simulink model "sm_pto_shaft"  (R2021b)
settings: Solver=ode15s  StartTime=0.0  StopTime=20  MaxStep=0.01  RelTol=1e-6  EnableMultiTasking=on
model workspace: external: MATLAB File sm_pto_shaft_params.m (data not in the file)
undefined symbols (not defined in the file or in its folder): actuator, clamp, linkage, plate, sigbuilder_block, sleeve, X, Y, Z
libraries: sm_lib x147, nesl_utility x8, simulink x1
(part 1 of 4)
Description:
  | Modeling Constant Velocity Joints - PTO Shaft
  | 
  | This example shows a Power Take-Off (PTO) shaft, a device for transferring
  | power from tractor engines to auxiliary equipment such as soil tillers
  | and wood chippers. The model includes two PTO subsystems identical in
  | every sense but their joints. One contains universal (U) joints, the
  | other constant-velocity (CV) joints.
  | 
  | At large bend angles, U joints lead to uneven rotations, subjecting the
  | adjoining shafts to relatively large vibrations and elevated internal
  | stresses. CV joints eliminate these by allowing the shafts to spin at
  | constant velocity, resulting in a smooth motion profile no matter the
  | bend angle.
  | 
  | A single set of motion inputs governs the behavior of the PTO subsystems.
  | The Scope block plots the resulting angular velocities and bend angles of
  | the shafts, enabling you to compare the kinematics of the two joint
  | types.
settings Model: Creator=The MathWorks, Inc.  LastModifiedBy=The MathWorks, Inc.
settings SolverCC: AlgebraicLoopSolver=TrustRegion
settings DataIOCC: LimitDataPoints=on  SaveFormat=Array  ReturnWorkspaceOutputs=off
settings OptimizationCC: LifeSpan=inf
settings DebuggingCC: SolverPrmCheckMsg=warning  SFUnexpectedBacktrackingDiag=warning  SFNoUnconditionalDefaultTransitionDiag=warning  SFExecutionAtInitializationDiag=none  SFMachineParentedDataDiag=warning  ArithmeticOperatorsInVariantConditions=warning
settings HardwareCC: ProdBitPerPointer=32  ProdBitPerSizeT=32  ProdBitPerPtrDiffT=32  ProdLargestAtomicFloat=None  ProdIntDivRoundTo=Undefined  ProdEndianess=Unspecified  ProdWordSize=32  ProdHWDeviceType=32-bit Generic
settings ModelReferenceCC: PropagateSignalLabelsOutOfModel=off
settings SFSimCC: SimUseLocalCustomCode=off  CustomCodeUndefinedFunction=UseInterfaceOnly
settings RTWCC: RTWUseLocalCustomCode=off
settings CodeAppCC: StateflowObjectComments=on
settings GRTTargetCC: TargetLangStandard=C89/C90 (ANSI)
settings ConfigComp: CovMetricSettings=dw  CovSaveCumulativeToWorkspaceVar=on  CovSaveSingleToWorkspaceVar=on  CovExternalEMLEnable=off  CovSFcnEnable=off
settings SimscapeCC: SimscapeNormalizeSystem=off
settings ConfigurationSet: Description=SimMechanics 2G
settings ExplorerConfigSet: InternalSimMechanicsExplorerSettings="<ExplorerConfiguration><canonicalview>default</canonicalview><AnimationSetting><BasePlaybackSpeed>1.0</BasePlaybackSpeed><PlaybackSpeedFactor>1.0</PlaybackSpeedFactor></AnimationSetting><TilePanel><TileInfo><Tiles Columns=\"1\" Count=\"1\" Rows=\"1\"><Column Left=\"2\" Weight=\"1\"/><Column Left=\"821\"/><Row Top=\"2\" Weight=\"1\"/><Row Top=\"584\"/><Tile Height=\"1\" Width=\"1\" X=\"0\" Y=\"0\"/></Tiles></TileInfo><SceneInfo><SceneViewer><BGColor><R>0.60000002384185791</R><G>0.60000002384185791</G><B>0.60000002384185791</B></BGColor><Camera><Position><X>2.5733745767261142</X><Y>-4.7840428425456913</Y><Z>3.9735506250049228</Z></Position><Center><X>-1.2699999809265137</X><Y>-0.94066828489303589</Y><Z>0.13017606735229492</Z></Center><Up><X>-0.40824829046386307</X><Y>0.40824829046386307</Y><Z>0.81649658092772615</Z></Up><Left>-2.0279375195503238</Left><Right>2.0279375195503238</Right><Bottom>-1.7125064849853517</Bottom><Top>1.7125064849853517</Top></Camera></SceneViewer></SceneInfo></TilePanel></ExplorerConfiguration>"

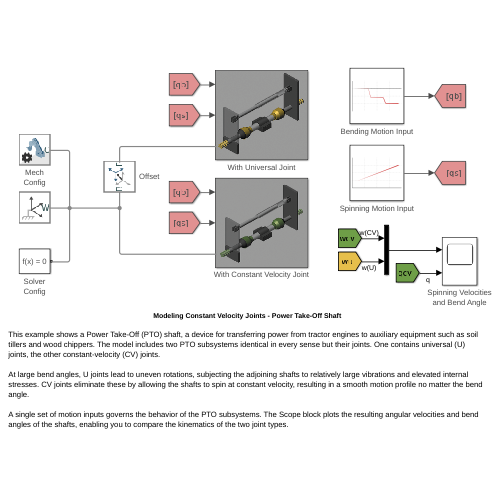
[thumbnail: Simulink's stored preview of the top-level diagram]
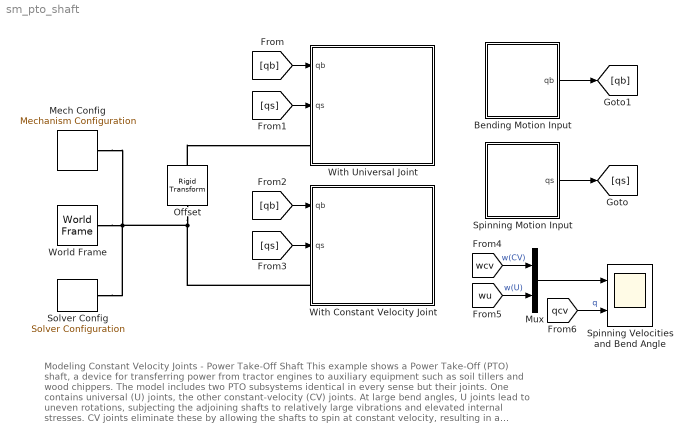
== system sm_pto_shaft ==
  note: Modeling Constant Velocity Joints - Power Take-Off Shaft
      |
      | This example shows a Power Take-Off (PTO) shaft, a device for transferring power from tractor engines to auxiliary equipment such as soil tillers and wood chippers. The model includes two PTO subsystems identical in every sense but their joints. One contains universal (U) joints, the other constant-velocity (CV) joints.
      |
      | At large bend angles, U joints lead to uneven rotations, subjecting the adjoining shafts to relatively large vibrations and elevated internal stresses. CV joints eliminate these by allowing the shafts to spin at constant velocity, resulting in a smooth motion profile no matter the bend angle.
      |
      | A single set of motion inputs governs the behavior of the PTO subsystems. The Scope block plots the resulting angular velocities and bend angles of the shafts, enabling you to compare the kinematics of the two joint types.
  Bending Motion Input : Subsystem
      mask Display: image(fullfile(matlabroot, 'toolbox', 'physmod', 'sm', 'smdemos', 'pto_shaft', 'images', 'bending_signal.svg'));
  Mech Config : sm_lib/Utilities/Mechanism Configuration  UniformGravity=None  GravityVector=[0 0 -9.80665]  GravityUnits=m/s^2  LinearizationDelta=0.001  JointModeTransitionNonlinearIterations=2
  Mux : Mux  Inputs=2
  Offset : sm_lib/Frames and Transforms/Rigid Transform  TranslationMethod=StandardAxis  TranslationStandardOffset=100  TranslationLengthUnit=in  TranslationStandardAxis=-X  TranslationCartesianOffset=[0 0 0]  TranslationROffset=0  TranslationROffsetUnits=m  TranslationZOffset=0  TranslationZOffsetUnits=m  TranslationThetaOffset=0  TranslationThetaOffsetUnits=deg  RotationMethod=None  RotationAngleUnits=deg  RotationStandardAxis=+X  RotationAngle=90  RotationArbitraryAxis=[0 0 1]  FollAlignAxisA=+X  BaseAlignAxisA=+Y  FollAlignAxisB=+Y  BaseAlignAxisB=+Z  RotationSequenceAxes=FollowerAxes  RotationSequence=XYX  RotationSequenceAngles=[0 0 0]  RotationSequenceAnglesUnits=deg  RotationMatrix=[1 0 0; 0 1 0; 0 0 1]
  Solver Config : nesl_utility/Solver Configuration  PhysicalDomain=network_engine_domain  SubClassName=solver  LeftPortType=input  RightPortType=generic  Tones=[]  Harmonics=[]  SimulateNoise=off  Profile=off  UseLocalSampling=off  EnableSwitchedLinearOptims=on  FrequencyDomain=off  UseCCode=off  RelTol=0.001  AbsTol=1e-06  MinStep=1e-09  ToWorkspace=off  RevertToSquareIcSolve=off  NumHomotopyIterations=100  PhasorMode=off  PhasorModeNumHarmonics=1  DoDC=off  ResidualTolerance=1e-09  UseLocalSolver=off  LocalSolverChoice=NE_BACKWARD_EULER_ADVANCER  LocalSolverSampleTime=0.001  DoFixedCost=off  MaxNonlinIter=3  MaxModeIter=2  ComputeImpulses=off  ImpulseIterations=2  LinearAlgebra=Sparse  EquationFormulation=NE_TIME_EF  DelaysMemoryBudget=1024  AutomaticFiltering=on  FilteringTimeConstant=0.001  PartitionStorageMethod=AS_NEEDED  PartitionMemoryBudget=1024  PartitionMethod=FAST
      settings: SourceProductBaseCode=PW,SS
  Spinning Motion Input : Subsystem
      mask Display: image(fullfile(matlabroot, 'toolbox', 'physmod', 'sm', 'smdemos', 'pto_shaft', 'images', 'spinning_ramp.svg'))
  Spinning Velocities and Bend Angle : Scope  NumInputPorts=2
  With Constant Velocity Joint : Subsystem
      mask Display: image(fullfile(matlabroot, 'toolbox', 'physmod', 'sm', 'smdemos', 'pto_shaft', 'images', 'cvj_pto.svg'));
  With Universal Joint : Subsystem
      mask Display: image(fullfile(matlabroot, 'toolbox', 'physmod', 'sm', 'smdemos', 'pto_shaft', 'images', 'uj_pto.svg'));
  World Frame : sm_lib/Frames and Transforms/World Frame
  wires:
  Bending Motion Input/1(qb) -> [qb]
  Spinning Motion Input/1(qs) -> [qs]
  [qb] -> With Constant Velocity Joint/1(qb)
  [qs] -> With Constant Velocity Joint/2(qs)
  [wcv] -> Mux/1  "w(CV)"
  [wu] -> Mux/2  "w(U)"
  Mux/1 -> Spinning Velocities and Bend Angle/1
  [qcv] -> Spinning Velocities and Bend Angle/2  "q"
  [qb] -> With Universal Joint/1(qb)
  [qs] -> With Universal Joint/2(qs)
  connections:
  Offset/RConn1 -- With Universal Joint/LConn1
  Offset/LConn1 -- With Constant Velocity Joint/LConn1 -- Mech Config/RConn1 -- Solver Config/RConn1 -- World Frame/RConn1

== system sm_pto_shaft/Bending Motion Input ==
  Gain : Gain  Gain=14.25
  Nondimensional Actuator Stroke : Subsystem  Tag=STV Subsys  LoadFcn=sigbuilder_block('load');  StartFcn=sigbuilder_block('start');  StopFcn=sigbuilder_block('stop');  ClipboardFcn=sigbuilder_block('clipboard');  mask(Sigbuilder block){tuvar=[0:10]}
      mask help: Simulink:masks:SigbuilderBlock_MD
      mask init:
      | if ~strcmp(get_param(bdroot(gcbh),'SimulationStatus'),'stopped') tuvar = sigbuilder_block('maskInit'); end
      settings: CopyFcn=sigbuilder_block('copy');  DeleteFcn=sigbuilder_block('delete');  ModelCloseFcn=sigbuilder_block('modelClose');  PreSaveFcn=sigbuilder_block('preSave');  PauseFcn=sigbuilder_block('pause');  ContinueFcn=sigbuilder_block('continue');  NameChangeFcn=sigbuilder_block('namechange');  OpenFcn=sigbuilder_block('open',[437.6 199.2 550.4 400 ]);  CloseFcn=sigbuilder_block('close');
      mask Display: plot(0, 0, 100, 100,[2, 2, 32, 32, 2], [68, 8, 8, 68, 68],[32, 2], [38, 38], [32, 19, 2],[53, 60, 44], [32, 17, 17, 2],[16, 16, 31, 31]);txt = getActiveGroup(gcbh);text(2, 100, txt,'verticalAlignment', 'top');
  qb : Outport  VectorParamsAs1DForOutWhenUnconnected=off
  wires:
  Gain/1 -> qb/1
  Nondimensional Actuator Stroke/1(Signal 1) -> Gain/1

== system sm_pto_shaft/Spinning Motion Input ==
  Gain : Gain  Gain=180
  Shaft Rotation : simulink/Sources/Ramp  slope=1  start=1  InitialOutput=0
  qs : Outport  VectorParamsAs1DForOutWhenUnconnected=off
  wires:
  Gain/1 -> qs/1
  Shaft Rotation/1 -> Gain/1

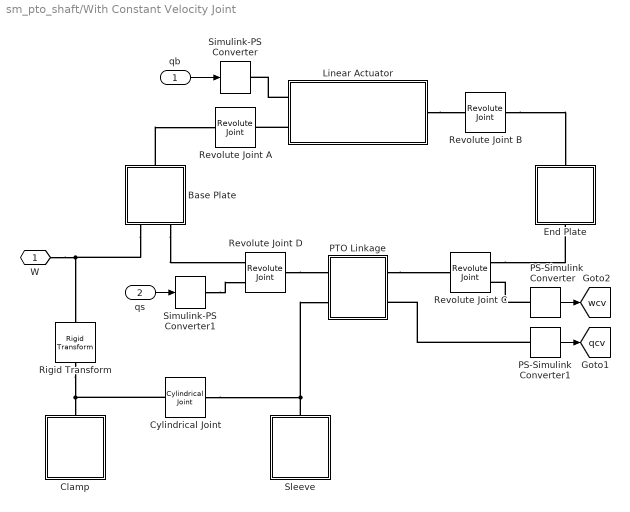
== system sm_pto_shaft/With Constant Velocity Joint ==
  qb : Inport
  qs : Inport  Port=2
  Base Plate : Subsystem  mask(Base Plate){hp=plate.height, wp=plate.width, tp=plate.thickness, R=plate.hole.radius, Lb=plate.bracket.length, wb=plate.bracket.width, tb=plate.bracket.thickness, Ri=plate.bracket.hole.radius, rgb=plate.color, alpha=plate.opacity, rho=plate.density}
      mask prompts: hp "Height (in)"; wp "Width (in)"; tp "Thickness (in)"; R "Hole Radius (in)"; Lb "Length (in)"; wb "Width (in)"; tb "Thickness (in)"; Ri "Inner Radius (in)"; rgb "Color (RGB)"; alpha "Opacity (unitless)"; rho "Density (kg/m^3)"
      mask help: This block models the fixed base plate supporting the PTO linkage.
      mask init:
      | % Plate cross-section coordinates:
      | theta = linspace(0, -pi)';
      | plateBottomCS = [-wp/2 -hp/4; wp/2 -hp/4; wp/2 0; R*cos(theta) R*sin(theta); -wp/2 0];
      | theta = linspace(pi, 0)';
      | plateTopCS = [-wp/2 0; R*cos(theta) R*sin(theta); wp/2 0; wp/2 3*hp/4; -wp/2 3*hp/4];
      | 
      | % Bracket cross-section coordinates:
      | Ro = wb/2;
      | theta = linspace(3*pi/2, pi/2)';
      | bracketBottomCS = [0 wb/2; -Lb wb/2; -Lb -wb/2; 0 -wb/2; Ri*cos(theta) Ri*sin(theta)];
      | thetaA = linspace(-pi/2, pi/2)';
      | betaB = linspace(pi/2, -pi/2)';
      | bracketTopCS = [Ro*cos(thetaA) Ro*sin(thetaA); Ri*cos(betaB) Ri*sin(betaB)];
      mask DialogControl Container19 Prompt: Plate
      mask DialogControl Container15 Prompt: Bracket
      mask DialogControl Container16 Prompt: Material Properties
      mask Display: image(fullfile(matlabroot, 'toolbox', 'physmod', 'sm', 'smdemos', 'pto_shaft', 'images', 'base.png'));
  Clamp : Subsystem  mask(Clamp){L=clamp.length, T=clamp.thickness, R=clamp.radius, D=clamp.wing.width, rgbClamp=clamp.color, rho=clamp.density}
      mask prompts: L "Length (in)"; T "Wall Thickness (in)"; R "Hole Radius (in)"; D "Wing Width (in)"; rgbClamp "Color (RGB)"; rho "Density (kg/m^3)"
      mask help: This block models a clamp used to hold the central shaft of the PTO linkage fixed.
      mask init:
      | % Common Parameters
      | HW = R+T+D; % Clamp Half Width
      | Ro = R + T; % Outer Clamp Radius
      | 
      | % Bottom Half CS
      | theta = linspace(0, -pi)';
      | bottomCS = [-HW -Ro; HW -Ro; HW 0; ...
      |     R*cos(theta) R*sin(theta); -HW 0];
      | 
      | % Top Half CS
      | theta = linspace(pi, 0)';
      | alpha = linspace(asin(T/Ro), pi-asin(T/Ro))';
      | topCS = [-HW 0; R*cos(theta) R*sin(theta); HW 0; HW T; ...
      |     Ro*cos(alpha) Ro*sin(alpha); -HW T];
      mask Display: image(fullfile(matlabroot, 'toolbox', 'physmod', 'sm', 'smdemos', 'pto_shaft', 'images', 'clamp.png'));
  Cylindrical Joint : sm_lib/Joints/Cylindrical Joint  JointMode=Normal  SenseConstraintForce=off  SenseConstraintForceX=off  SenseConstraintForceY=off  SenseConstraintForceZ=off  SenseConstraintTorque=off  SenseConstraintTorqueX=off  SenseConstraintTorqueY=off  SenseConstraintTorqueZ=off  SenseTotalForce=off  SenseTotalForceX=off  SenseTotalForceY=off  SenseTotalForceZ=off  SenseTotalTorque=off  SenseTotalTorqueX=off  SenseTotalTorqueY=off  SenseTotalTorqueZ=off  CompositeWrenchDir=FollowerOnBase  CompositeWrenchFrame=BaseFrame  PzEquilibriumPosition=0  PzEquilibriumPositionUnits=m  PzSpringStiffness=0  PzSpringStiffnessUnits=N/m  PzDampingCoefficient=0  PzDampingCoefficientUnits=N/(m/s)  PzTorqueActuationMode=NoTorque  PzMotionActuationMode=ComputedMotion  PzSensePosition=off  PzSenseVelocity=off  PzSenseAcceleration=off  PzSenseTorqueForce=off  PzSenseLowerLimitTorqueForce=off  PzSenseUpperLimitTorqueForce=off  PzLowerLimitSpecify=off  PzLowerLimitBound=-1  PzLowerLimitBoundUnits=m  PzLowerLimitStiffness=1e6  PzLowerLimitStiffnessUnits=N/m  PzLowerLimitDamping=1e3  PzLowerLimitDampingUnits=N/(m/s)  PzLowerLimitTransitionRegionWidth=1e-4  PzLowerLimitTransitionRegionWidthUnits=m  PzUpperLimitSpecify=off  PzUpperLimitBound=1  PzUpperLimitBoundUnits=m  PzUpperLimitStiffness=1e6  PzUpperLimitStiffnessUnits=N/m  PzUpperLimitDamping=1e3  PzUpperLimitDampingUnits=N/(m/s)  PzUpperLimitTransitionRegionWidth=1e-4  PzUpperLimitTransitionRegionWidthUnits=m  PzPositionTargetSpecify=off  PzPositionTargetPriority=High  PzPositionTargetValue=0  PzPositionTargetValueUnits=m  PzVelocityTargetSpecify=off  PzVelocityTargetPriority=High  PzVelocityTargetValue=0  PzVelocityTargetValueUnits=m/s  RzEquilibriumPosition=0  RzEquilibriumPositionUnits=deg  RzSpringStiffness=0  RzSpringStiffnessUnits=N*m/deg  RzDampingCoefficient=0  RzDampingCoefficientUnits=N*m/(deg/s)  RzTorqueActuationMode=NoTorque  RzMotionActuationMode=ComputedMotion  RzSensePosition=off  RzSenseVelocity=off  RzSenseAcceleration=off  RzSenseTorqueForce=off  RzSenseLowerLimitTorqueForce=off  RzSenseUpperLimitTorqueForce=off  RzLowerLimitSpecify=off  RzLowerLimitBound=-90  RzLowerLimitBoundUnits=deg  RzLowerLimitStiffness=1e4  RzLowerLimitStiffnessUnits=N*m/deg  RzLowerLimitDamping=10  RzLowerLimitDampingUnits=N*m/(deg/s)  RzLowerLimitTransitionRegionWidth=0.1  RzLowerLimitTransitionRegionWidthUnits=deg  RzUpperLimitSpecify=off  RzUpperLimitBound=90  RzUpperLimitBoundUnits=deg  RzUpperLimitStiffness=1e4  RzUpperLimitStiffnessUnits=N*m/deg  RzUpperLimitDamping=10  RzUpperLimitDampingUnits=N*m/(deg/s)  RzUpperLimitTransitionRegionWidth=0.1  RzUpperLimitTransitionRegionWidthUnits=deg  RzPositionTargetSpecify=off  RzPositionTargetPriority=High  RzPositionTargetValue=0  RzPositionTargetValueUnits=deg  RzVelocityTargetSpecify=off  RzVelocityTargetPriority=High  RzVelocityTargetValue=0  RzVelocityTargetValueUnits=deg/s
  End Plate : Subsystem  mask(End Plate){hp=plate.height, wp=plate.width, tp=plate.thickness, R=plate.hole.radius, Lb=plate.bracket.length, wb=plate.bracket.width, tb=plate.bracket.thickness, Ri=plate.bracket.hole.radius, rgb=plate.color, alpha=plate.opacity, rho=plate.density}
      mask prompts: hp "Height (in)"; wp "Width (in)"; tp "Thickness (in)"; R "Hole Radius (in)"; Lb "Length (in)"; wb "Width (in)"; tb "Thickness (in)"; Ri "Inner Radius (in)"; rgb "Color (RGB)"; alpha "Opacity (unitless)"; rho "Density (kg/m^3)"
      mask help: This block models the tilting end plate supporting the PTO linkage.
      mask init: same as sm_pto_shaft/With Constant Velocity Joint/Base Plate
      mask DialogControl Container19 Prompt: Plate
      mask DialogControl Container15 Prompt: Bracket
      mask DialogControl Container16 Prompt: Material Properties
      mask Display: image(fullfile(matlabroot, 'toolbox', 'physmod', 'sm', 'smdemos', 'pto_shaft', 'images', 'base.png'));
  Linear Actuator : Subsystem
      mask Display: image(fullfile(matlabroot, 'toolbox', 'physmod', 'sm', 'smdemos', 'pto_shaft', 'images', 'linear_actuator.png'));
  PS-Simulink Converter : nesl_utility/PS-Simulink Converter  PhysicalDomain=network_engine_domain  SubClassName=ps_output  LeftPortType=input  RightPortType=output  PseudoPeriodic=off  Frequencies=[]  Unit=deg/s  AffineConversion=off
      settings: SourceProductBaseCode=PW,SS
  PS-Simulink Converter1 : nesl_utility/PS-Simulink Converter  PhysicalDomain=network_engine_domain  SubClassName=ps_output  LeftPortType=input  RightPortType=output  PseudoPeriodic=off  Frequencies=[]  Unit=deg  AffineConversion=off
      settings: SourceProductBaseCode=PW,SS
  PTO Linkage : Subsystem
      mask Display: image(fullfile(matlabroot, 'toolbox', 'physmod', 'sm', 'smdemos', 'pto_shaft', 'images', 'pto_linkage.png'));
  Revolute Joint A : sm_lib/Joints/Revolute Joint  JointMode=Normal  SenseConstraintForce=off  SenseConstraintForceX=off  SenseConstraintForceY=off  SenseConstraintForceZ=off  SenseConstraintTorque=off  SenseConstraintTorqueX=off  SenseConstraintTorqueY=off  SenseConstraintTorqueZ=off  SenseTotalForce=off  SenseTotalForceX=off  SenseTotalForceY=off  SenseTotalForceZ=off  SenseTotalTorque=off  SenseTotalTorqueX=off  SenseTotalTorqueY=off  SenseTotalTorqueZ=off  CompositeWrenchDir=FollowerOnBase  CompositeWrenchFrame=BaseFrame  EquilibriumPosition=0  EquilibriumPositionUnits=deg  SpringStiffness=0  SpringStiffnessUnits=N*m/deg  DampingCoefficient=0  DampingCoefficientUnits=N*m/(deg/s)  TorqueActuationMode=NoTorque  MotionActuationMode=ComputedMotion  SensePosition=off  SenseVelocity=off  SenseAcceleration=off  SenseTorqueForce=off  SenseLowerLimitTorqueForce=off  SenseUpperLimitTorqueForce=off  LowerLimitSpecify=off  LowerLimitBound=-90  LowerLimitBoundUnits=deg  LowerLimitStiffness=1e4  LowerLimitStiffnessUnits=N*m/deg  LowerLimitDamping=10  LowerLimitDampingUnits=N*m/(deg/s)  LowerLimitTransitionRegionWidth=0.1  LowerLimitTransitionRegionWidthUnits=deg  UpperLimitSpecify=off  UpperLimitBound=90  UpperLimitBoundUnits=deg  UpperLimitStiffness=1e4  UpperLimitStiffnessUnits=N*m/deg  UpperLimitDamping=10  UpperLimitDampingUnits=N*m/(deg/s)  UpperLimitTransitionRegionWidth=0.1  UpperLimitTransitionRegionWidthUnits=deg  PositionTargetSpecify=off  PositionTargetPriority=High  PositionTargetValue=0  PositionTargetValueUnits=deg  VelocityTargetSpecify=off  VelocityTargetPriority=High  VelocityTargetValue=0  VelocityTargetValueUnits=deg/s
  Revolute Joint B : sm_lib/Joints/Revolute Joint  JointMode=Normal  SenseConstraintForce=off  SenseConstraintForceX=off  SenseConstraintForceY=off  SenseConstraintForceZ=off  SenseConstraintTorque=off  SenseConstraintTorqueX=off  SenseConstraintTorqueY=off  SenseConstraintTorqueZ=off  SenseTotalForce=off  SenseTotalForceX=off  SenseTotalForceY=off  SenseTotalForceZ=off  SenseTotalTorque=off  SenseTotalTorqueX=off  SenseTotalTorqueY=off  SenseTotalTorqueZ=off  CompositeWrenchDir=FollowerOnBase  CompositeWrenchFrame=BaseFrame  EquilibriumPosition=0  EquilibriumPositionUnits=deg  SpringStiffness=0  SpringStiffnessUnits=N*m/deg  DampingCoefficient=0  DampingCoefficientUnits=N*m/(deg/s)  TorqueActuationMode=NoTorque  MotionActuationMode=ComputedMotion  SensePosition=off  SenseVelocity=off  SenseAcceleration=off  SenseTorqueForce=off  SenseLowerLimitTorqueForce=off  SenseUpperLimitTorqueForce=off  LowerLimitSpecify=off  LowerLimitBound=-90  LowerLimitBoundUnits=deg  LowerLimitStiffness=1e4  LowerLimitStiffnessUnits=N*m/deg  LowerLimitDamping=10  LowerLimitDampingUnits=N*m/(deg/s)  LowerLimitTransitionRegionWidth=0.1  LowerLimitTransitionRegionWidthUnits=deg  UpperLimitSpecify=off  UpperLimitBound=90  UpperLimitBoundUnits=deg  UpperLimitStiffness=1e4  UpperLimitStiffnessUnits=N*m/deg  UpperLimitDamping=10  UpperLimitDampingUnits=N*m/(deg/s)  UpperLimitTransitionRegionWidth=0.1  UpperLimitTransitionRegionWidthUnits=deg  PositionTargetSpecify=off  PositionTargetPriority=High  PositionTargetValue=0  PositionTargetValueUnits=deg  VelocityTargetSpecify=off  VelocityTargetPriority=High  VelocityTargetValue=0  VelocityTargetValueUnits=deg/s
  Revolute Joint C : sm_lib/Joints/Revolute Joint  JointMode=Normal  SenseConstraintForce=off  SenseConstraintForceX=off  SenseConstraintForceY=off  SenseConstraintForceZ=off  SenseConstraintTorque=off  SenseConstraintTorqueX=off  SenseConstraintTorqueY=off  SenseConstraintTorqueZ=off  SenseTotalForce=off  SenseTotalForceX=off  SenseTotalForceY=off  SenseTotalForceZ=off  SenseTotalTorque=off  SenseTotalTorqueX=off  SenseTotalTorqueY=off  SenseTotalTorqueZ=off  CompositeWrenchDir=FollowerOnBase  CompositeWrenchFrame=BaseFrame  EquilibriumPosition=0  EquilibriumPositionUnits=deg  SpringStiffness=0  SpringStiffnessUnits=N*m/deg  DampingCoefficient=0  DampingCoefficientUnits=N*m/(deg/s)  TorqueActuationMode=NoTorque  MotionActuationMode=ComputedMotion  SensePosition=off  SenseVelocity=on  SenseAcceleration=off  SenseTorqueForce=off  SenseLowerLimitTorqueForce=off  SenseUpperLimitTorqueForce=off  LowerLimitSpecify=off  LowerLimitBound=-90  LowerLimitBoundUnits=deg  LowerLimitStiffness=1e4  LowerLimitStiffnessUnits=N*m/deg  LowerLimitDamping=10  LowerLimitDampingUnits=N*m/(deg/s)  LowerLimitTransitionRegionWidth=0.1  LowerLimitTransitionRegionWidthUnits=deg  UpperLimitSpecify=off  UpperLimitBound=90  UpperLimitBoundUnits=deg  UpperLimitStiffness=1e4  UpperLimitStiffnessUnits=N*m/deg  UpperLimitDamping=10  UpperLimitDampingUnits=N*m/(deg/s)  UpperLimitTransitionRegionWidth=0.1  UpperLimitTransitionRegionWidthUnits=deg  PositionTargetSpecify=off  PositionTargetPriority=High  PositionTargetValue=0  PositionTargetValueUnits=deg  VelocityTargetSpecify=off  VelocityTargetPriority=High  VelocityTargetValue=0  VelocityTargetValueUnits=deg/s
  Revolute Joint D : sm_lib/Joints/Revolute Joint  JointMode=Normal  SenseConstraintForce=off  SenseConstraintForceX=off  SenseConstraintForceY=off  SenseConstraintForceZ=off  SenseConstraintTorque=off  SenseConstraintTorqueX=off  SenseConstraintTorqueY=off  SenseConstraintTorqueZ=off  SenseTotalForce=off  SenseTotalForceX=off  SenseTotalForceY=off  SenseTotalForceZ=off  SenseTotalTorque=off  SenseTotalTorqueX=off  SenseTotalTorqueY=off  SenseTotalTorqueZ=off  CompositeWrenchDir=FollowerOnBase  CompositeWrenchFrame=BaseFrame  EquilibriumPosition=0  EquilibriumPositionUnits=deg  SpringStiffness=0  SpringStiffnessUnits=N*m/deg  DampingCoefficient=0  DampingCoefficientUnits=N*m/(deg/s)  TorqueActuationMode=ComputedTorque  MotionActuationMode=InputMotion  SensePosition=off  SenseVelocity=off  SenseAcceleration=off  SenseTorqueForce=off  SenseLowerLimitTorqueForce=off  SenseUpperLimitTorqueForce=off  LowerLimitSpecify=off  LowerLimitBound=-90  LowerLimitBoundUnits=deg  LowerLimitStiffness=1e4  LowerLimitStiffnessUnits=N*m/deg  LowerLimitDamping=10  LowerLimitDampingUnits=N*m/(deg/s)  LowerLimitTransitionRegionWidth=0.1  LowerLimitTransitionRegionWidthUnits=deg  UpperLimitSpecify=off  UpperLimitBound=90  UpperLimitBoundUnits=deg  UpperLimitStiffness=1e4  UpperLimitStiffnessUnits=N*m/deg  UpperLimitDamping=10  UpperLimitDampingUnits=N*m/(deg/s)  UpperLimitTransitionRegionWidth=0.1  UpperLimitTransitionRegionWidthUnits=deg  PositionTargetSpecify=off  PositionTargetPriority=High  PositionTargetValue=0  PositionTargetValueUnits=deg  VelocityTargetSpecify=off  VelocityTargetPriority=High  VelocityTargetValue=0  VelocityTargetValueUnits=deg/s
  Rigid Transform : sm_lib/Frames and Transforms/Rigid Transform  TranslationMethod=StandardAxis  TranslationStandardOffset=34  TranslationLengthUnit=in  TranslationStandardAxis=-Y  TranslationCartesianOffset=[0 0 0]  TranslationROffset=0  TranslationROffsetUnits=m  TranslationZOffset=0  TranslationZOffsetUnits=m  TranslationThetaOffset=0  TranslationThetaOffsetUnits=deg  RotationMethod=StandardAxis  RotationAngleUnits=deg  RotationStandardAxis=+X  RotationAngle=90  RotationArbitraryAxis=[0 0 1]  FollAlignAxisA=+X  BaseAlignAxisA=+Y  FollAlignAxisB=+Y  BaseAlignAxisB=+Z  RotationSequenceAxes=FollowerAxes  RotationSequence=XYX  RotationSequenceAngles=[0 0 0]  RotationSequenceAnglesUnits=deg  RotationMatrix=[1 0 0; 0 1 0; 0 0 1]
  Simulink-PS Converter : nesl_utility/Simulink-PS Converter  PhysicalDomain=network_engine_domain  SubClassName=ps_input  LeftPortType=input  RightPortType=output  PseudoPeriodic=off  Frequencies=[]  NoiseDistribution=none  NoiseParameters=[]  Unit=in  AffineConversion=off  FilteringAndDerivatives=filter  SimscapeFilterOrder=2  InputFilterTimeConstant=0.1  UdotUserProvided=1
      settings: SourceProductBaseCode=PW,SS
  Simulink-PS Converter1 : nesl_utility/Simulink-PS Converter  PhysicalDomain=network_engine_domain  SubClassName=ps_input  LeftPortType=input  RightPortType=output  PseudoPeriodic=off  Frequencies=[]  NoiseDistribution=none  NoiseParameters=[]  Unit=deg  AffineConversion=off  FilteringAndDerivatives=filter  SimscapeFilterOrder=2  InputFilterTimeConstant=0.01  UdotUserProvided=1
      settings: SourceProductBaseCode=PW,SS
  Sleeve : Subsystem  mask(Sleeve){L=sleeve.length, R=sleeve.radius, t=sleeve.thickness, rgbShaft=sleeve.colorA, rgbBoot=sleeve.colorCVJ, rho=sleeve.density}
      mask prompts: L "Shaft Length (in)"; R "Shaft Radius (in)"; t "Shaft Thickness (in)"; rgbShaft "Shaft Color (RGB)"; rgbBoot "Boot Color (RGB)"; rho "Density (kg/m^3)"
      mask help: This block models a sleeve covering the central shaft of the PTO linkage.
      mask init:
      | bootCS = [2.77 0;2.77 0.22;2.66 0.22;2.66 2.33;3.33 2.33;4.55 4.77;4.77 9.5;4.22 4.77;3.11 2.66;2.44 2.66;2.44 0.33;1.44 0.33;1.44 0];
      | shaftCS = [(R-t) -L/2; R -L/2; R L/2; (R-t) L/2];
      mask Display: image(fullfile(matlabroot, 'toolbox', 'physmod', 'sm', 'smdemos', 'pto_shaft', 'images', 'cvj_sleeve.png'));
  W : PMIOPort  Side=Left
  tag scope: qcv=global, wcv=global
  wires:
  qb/1 -> Simulink-PS Converter/1
  qs/1 -> Simulink-PS Converter1/1
  PS-Simulink Converter/1 -> [wcv]
  PS-Simulink Converter1/1 -> [qcv]
  connections:
  Linear Actuator/LConn1 -- Simulink-PS Converter/RConn1
  Rigid Transform/RConn1 -- Clamp/RConn1 -- Cylindrical Joint/LConn1
  W/RConn1 -- Base Plate/LConn1 -- Rigid Transform/LConn1
  Sleeve/LConn1 -- PTO Linkage/RConn2 -- Cylindrical Joint/RConn1
  Linear Actuator/RConn1 -- Revolute Joint B/LConn1
  Linear Actuator/LConn2 -- Revolute Joint A/RConn1
  Simulink-PS Converter1/RConn1 -- Revolute Joint D/LConn2
  PS-Simulink Converter/LConn1 -- Revolute Joint C/RConn2
  Revolute Joint C/RConn1 -- End Plate/LConn1
  Revolute Joint B/RConn1 -- End Plate/RConn1
  Base Plate/RConn1 -- Revolute Joint A/LConn1
  Base Plate/LConn2 -- Revolute Joint D/LConn1
  Revolute Joint D/RConn1 -- PTO Linkage/RConn1
  PTO Linkage/LConn1 -- Revolute Joint C/LConn1
  PS-Simulink Converter1/LConn1 -- PTO Linkage/LConn2

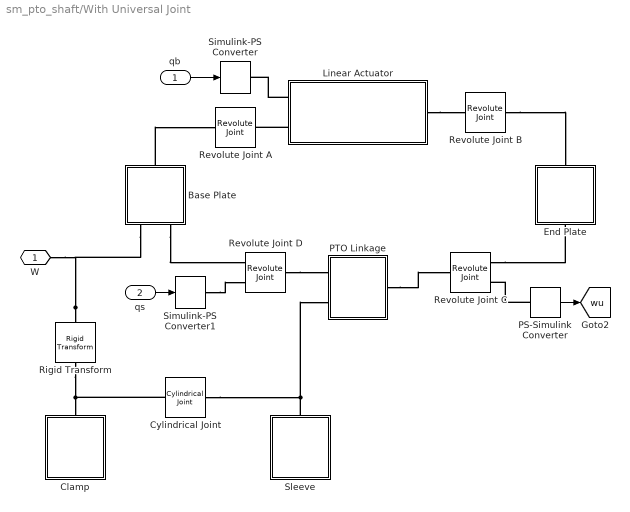
== system sm_pto_shaft/With Universal Joint ==
  qb : Inport
  qs : Inport  Port=2
  Base Plate : Subsystem  mask(Base Plate){hp=plate.height, wp=plate.width, tp=plate.thickness, R=plate.hole.radius, Lb=plate.bracket.length, wb=plate.bracket.width, tb=plate.bracket.thickness, Ri=plate.bracket.hole.radius, rgb=plate.color, alpha=plate.opacity, rho=plate.density}
      mask prompts: hp "Height (in)"; wp "Width (in)"; tp "Thickness (in)"; R "Hole Radius (in)"; Lb "Length (in)"; wb "Width (in)"; tb "Thickness (in)"; Ri "Inner Radius (in)"; rgb "Color (RGB)"; alpha "Opacity (unitless)"; rho "Density (kg/m^3)"
      mask help: This block models the fixed base plate supporting the PTO linkage.
      mask init: same as sm_pto_shaft/With Constant Velocity Joint/Base Plate
      mask DialogControl Container19 Prompt: Plate
      mask DialogControl Container15 Prompt: Bracket
      mask DialogControl Container16 Prompt: Material Properties
      mask Display: image(fullfile(matlabroot, 'toolbox', 'physmod', 'sm', 'smdemos', 'pto_shaft', 'images', 'base.png'));
  Clamp : Subsystem  mask(Clamp){L=clamp.length, T=clamp.thickness, R=clamp.radius, D=clamp.wing.width, rgbClamp=clamp.color, rho=clamp.density}
      mask prompts: L "Length (in)"; T "Wall Thickness (in)"; R "Hole Radius (in)"; D "Wing Width (in)"; rgbClamp "Color (RGB)"; rho "Density (kg/m^3)"
      mask help: This block models a clamp used to hold the central shaft of the PTO linkage fixed.
      mask init: same as sm_pto_shaft/With Constant Velocity Joint/Clamp
      mask Display: image(fullfile(matlabroot, 'toolbox', 'physmod', 'sm', 'smdemos', 'pto_shaft', 'images', 'clamp.png'));
  Cylindrical Joint : sm_lib/Joints/Cylindrical Joint  JointMode=Normal  SenseConstraintForce=off  SenseConstraintForceX=off  SenseConstraintForceY=off  SenseConstraintForceZ=off  SenseConstraintTorque=off  SenseConstraintTorqueX=off  SenseConstraintTorqueY=off  SenseConstraintTorqueZ=off  SenseTotalForce=off  SenseTotalForceX=off  SenseTotalForceY=off  SenseTotalForceZ=off  SenseTotalTorque=off  SenseTotalTorqueX=off  SenseTotalTorqueY=off  SenseTotalTorqueZ=off  CompositeWrenchDir=FollowerOnBase  CompositeWrenchFrame=BaseFrame  PzEquilibriumPosition=0  PzEquilibriumPositionUnits=m  PzSpringStiffness=0  PzSpringStiffnessUnits=N/m  PzDampingCoefficient=0  PzDampingCoefficientUnits=N/(m/s)  PzTorqueActuationMode=NoTorque  PzMotionActuationMode=ComputedMotion  PzSensePosition=off  PzSenseVelocity=off  PzSenseAcceleration=off  PzSenseTorqueForce=off  PzSenseLowerLimitTorqueForce=off  PzSenseUpperLimitTorqueForce=off  PzLowerLimitSpecify=off  PzLowerLimitBound=-1  PzLowerLimitBoundUnits=m  PzLowerLimitStiffness=1e6  PzLowerLimitStiffnessUnits=N/m  PzLowerLimitDamping=1e3  PzLowerLimitDampingUnits=N/(m/s)  PzLowerLimitTransitionRegionWidth=1e-4  PzLowerLimitTransitionRegionWidthUnits=m  PzUpperLimitSpecify=off  PzUpperLimitBound=1  PzUpperLimitBoundUnits=m  PzUpperLimitStiffness=1e6  PzUpperLimitStiffnessUnits=N/m  PzUpperLimitDamping=1e3  PzUpperLimitDampingUnits=N/(m/s)  PzUpperLimitTransitionRegionWidth=1e-4  PzUpperLimitTransitionRegionWidthUnits=m  PzPositionTargetSpecify=off  PzPositionTargetPriority=High  PzPositionTargetValue=0  PzPositionTargetValueUnits=m  PzVelocityTargetSpecify=off  PzVelocityTargetPriority=High  PzVelocityTargetValue=0  PzVelocityTargetValueUnits=m/s  RzEquilibriumPosition=0  RzEquilibriumPositionUnits=deg  RzSpringStiffness=0  RzSpringStiffnessUnits=N*m/deg  RzDampingCoefficient=0  RzDampingCoefficientUnits=N*m/(deg/s)  RzTorqueActuationMode=NoTorque  RzMotionActuationMode=ComputedMotion  RzSensePosition=off  RzSenseVelocity=off  RzSenseAcceleration=off  RzSenseTorqueForce=off  RzSenseLowerLimitTorqueForce=off  RzSenseUpperLimitTorqueForce=off  RzLowerLimitSpecify=off  RzLowerLimitBound=-90  RzLowerLimitBoundUnits=deg  RzLowerLimitStiffness=1e4  RzLowerLimitStiffnessUnits=N*m/deg  RzLowerLimitDamping=10  RzLowerLimitDampingUnits=N*m/(deg/s)  RzLowerLimitTransitionRegionWidth=0.1  RzLowerLimitTransitionRegionWidthUnits=deg  RzUpperLimitSpecify=off  RzUpperLimitBound=90  RzUpperLimitBoundUnits=deg  RzUpperLimitStiffness=1e4  RzUpperLimitStiffnessUnits=N*m/deg  RzUpperLimitDamping=10  RzUpperLimitDampingUnits=N*m/(deg/s)  RzUpperLimitTransitionRegionWidth=0.1  RzUpperLimitTransitionRegionWidthUnits=deg  RzPositionTargetSpecify=off  RzPositionTargetPriority=High  RzPositionTargetValue=0  RzPositionTargetValueUnits=deg  RzVelocityTargetSpecify=off  RzVelocityTargetPriority=High  RzVelocityTargetValue=0  RzVelocityTargetValueUnits=deg/s
  End Plate : Subsystem  mask(End Plate){hp=plate.height, wp=plate.width, tp=plate.thickness, R=plate.hole.radius, Lb=plate.bracket.length, wb=plate.bracket.width, tb=plate.bracket.thickness, Ri=plate.bracket.hole.radius, rgb=plate.color, alpha=plate.opacity, rho=plate.density}
      mask prompts: hp "Height (in)"; wp "Width (in)"; tp "Thickness (in)"; R "Hole Radius (in)"; Lb "Length (in)"; wb "Width (in)"; tb "Thickness (in)"; Ri "Inner Radius (in)"; rgb "Color (RGB)"; alpha "Opacity (unitless)"; rho "Density (kg/m^3)"
      mask help: This block models the tilting end plate supporting the PTO linkage.
      mask init: same as sm_pto_shaft/With Constant Velocity Joint/Base Plate
      mask DialogControl Container19 Prompt: Plate
      mask DialogControl Container15 Prompt: Bracket
      mask DialogControl Container16 Prompt: Material Properties
      mask Display: image(fullfile(matlabroot, 'toolbox', 'physmod', 'sm', 'smdemos', 'pto_shaft', 'images', 'base.png'));
  Linear Actuator : Subsystem
      mask Display: image(fullfile(matlabroot, 'toolbox', 'physmod', 'sm', 'smdemos', 'pto_shaft', 'images', 'linear_actuator.png'));
  PS-Simulink Converter : nesl_utility/PS-Simulink Converter  PhysicalDomain=network_engine_domain  SubClassName=ps_output  LeftPortType=input  RightPortType=output  PseudoPeriodic=off  Frequencies=[]  Unit=deg/s  AffineConversion=off
      settings: SourceProductBaseCode=PW,SS
  PTO Linkage : Subsystem
      mask Display: image(fullfile(matlabroot, 'toolbox', 'physmod', 'sm', 'smdemos', 'pto_shaft', 'images', 'pto_linkage.png'));
  Revolute Joint A : sm_lib/Joints/Revolute Joint  JointMode=Normal  SenseConstraintForce=off  SenseConstraintForceX=off  SenseConstraintForceY=off  SenseConstraintForceZ=off  SenseConstraintTorque=off  SenseConstraintTorqueX=off  SenseConstraintTorqueY=off  SenseConstraintTorqueZ=off  SenseTotalForce=off  SenseTotalForceX=off  SenseTotalForceY=off  SenseTotalForceZ=off  SenseTotalTorque=off  SenseTotalTorqueX=off  SenseTotalTorqueY=off  SenseTotalTorqueZ=off  CompositeWrenchDir=FollowerOnBase  CompositeWrenchFrame=BaseFrame  EquilibriumPosition=0  EquilibriumPositionUnits=deg  SpringStiffness=0  SpringStiffnessUnits=N*m/deg  DampingCoefficient=0  DampingCoefficientUnits=N*m/(deg/s)  TorqueActuationMode=NoTorque  MotionActuationMode=ComputedMotion  SensePosition=off  SenseVelocity=off  SenseAcceleration=off  SenseTorqueForce=off  SenseLowerLimitTorqueForce=off  SenseUpperLimitTorqueForce=off  LowerLimitSpecify=off  LowerLimitBound=-90  LowerLimitBoundUnits=deg  LowerLimitStiffness=1e4  LowerLimitStiffnessUnits=N*m/deg  LowerLimitDamping=10  LowerLimitDampingUnits=N*m/(deg/s)  LowerLimitTransitionRegionWidth=0.1  LowerLimitTransitionRegionWidthUnits=deg  UpperLimitSpecify=off  UpperLimitBound=90  UpperLimitBoundUnits=deg  UpperLimitStiffness=1e4  UpperLimitStiffnessUnits=N*m/deg  UpperLimitDamping=10  UpperLimitDampingUnits=N*m/(deg/s)  UpperLimitTransitionRegionWidth=0.1  UpperLimitTransitionRegionWidthUnits=deg  PositionTargetSpecify=off  PositionTargetPriority=High  PositionTargetValue=0  PositionTargetValueUnits=deg  VelocityTargetSpecify=off  VelocityTargetPriority=High  VelocityTargetValue=0  VelocityTargetValueUnits=deg/s
  Revolute Joint B : sm_lib/Joints/Revolute Joint  JointMode=Normal  SenseConstraintForce=off  SenseConstraintForceX=off  SenseConstraintForceY=off  SenseConstraintForceZ=off  SenseConstraintTorque=off  SenseConstraintTorqueX=off  SenseConstraintTorqueY=off  SenseConstraintTorqueZ=off  SenseTotalForce=off  SenseTotalForceX=off  SenseTotalForceY=off  SenseTotalForceZ=off  SenseTotalTorque=off  SenseTotalTorqueX=off  SenseTotalTorqueY=off  SenseTotalTorqueZ=off  CompositeWrenchDir=FollowerOnBase  CompositeWrenchFrame=BaseFrame  EquilibriumPosition=0  EquilibriumPositionUnits=deg  SpringStiffness=0  SpringStiffnessUnits=N*m/deg  DampingCoefficient=0  DampingCoefficientUnits=N*m/(deg/s)  TorqueActuationMode=NoTorque  MotionActuationMode=ComputedMotion  SensePosition=off  SenseVelocity=off  SenseAcceleration=off  SenseTorqueForce=off  SenseLowerLimitTorqueForce=off  SenseUpperLimitTorqueForce=off  LowerLimitSpecify=off  LowerLimitBound=-90  LowerLimitBoundUnits=deg  LowerLimitStiffness=1e4  LowerLimitStiffnessUnits=N*m/deg  LowerLimitDamping=10  LowerLimitDampingUnits=N*m/(deg/s)  LowerLimitTransitionRegionWidth=0.1  LowerLimitTransitionRegionWidthUnits=deg  UpperLimitSpecify=off  UpperLimitBound=90  UpperLimitBoundUnits=deg  UpperLimitStiffness=1e4  UpperLimitStiffnessUnits=N*m/deg  UpperLimitDamping=10  UpperLimitDampingUnits=N*m/(deg/s)  UpperLimitTransitionRegionWidth=0.1  UpperLimitTransitionRegionWidthUnits=deg  PositionTargetSpecify=off  PositionTargetPriority=High  PositionTargetValue=0  PositionTargetValueUnits=deg  VelocityTargetSpecify=off  VelocityTargetPriority=High  VelocityTargetValue=0  VelocityTargetValueUnits=deg/s
  Revolute Joint C : sm_lib/Joints/Revolute Joint  JointMode=Normal  SenseConstraintForce=off  SenseConstraintForceX=off  SenseConstraintForceY=off  SenseConstraintForceZ=off  SenseConstraintTorque=off  SenseConstraintTorqueX=off  SenseConstraintTorqueY=off  SenseConstraintTorqueZ=off  SenseTotalForce=off  SenseTotalForceX=off  SenseTotalForceY=off  SenseTotalForceZ=off  SenseTotalTorque=off  SenseTotalTorqueX=off  SenseTotalTorqueY=off  SenseTotalTorqueZ=off  CompositeWrenchDir=FollowerOnBase  CompositeWrenchFrame=BaseFrame  EquilibriumPosition=0  EquilibriumPositionUnits=deg  SpringStiffness=0  SpringStiffnessUnits=N*m/deg  DampingCoefficient=0  DampingCoefficientUnits=N*m/(deg/s)  TorqueActuationMode=NoTorque  MotionActuationMode=ComputedMotion  SensePosition=off  SenseVelocity=on  SenseAcceleration=off  SenseTorqueForce=off  SenseLowerLimitTorqueForce=off  SenseUpperLimitTorqueForce=off  LowerLimitSpecify=off  LowerLimitBound=-90  LowerLimitBoundUnits=deg  LowerLimitStiffness=1e4  LowerLimitStiffnessUnits=N*m/deg  LowerLimitDamping=10  LowerLimitDampingUnits=N*m/(deg/s)  LowerLimitTransitionRegionWidth=0.1  LowerLimitTransitionRegionWidthUnits=deg  UpperLimitSpecify=off  UpperLimitBound=90  UpperLimitBoundUnits=deg  UpperLimitStiffness=1e4  UpperLimitStiffnessUnits=N*m/deg  UpperLimitDamping=10  UpperLimitDampingUnits=N*m/(deg/s)  UpperLimitTransitionRegionWidth=0.1  UpperLimitTransitionRegionWidthUnits=deg  PositionTargetSpecify=off  PositionTargetPriority=High  PositionTargetValue=0  PositionTargetValueUnits=deg  VelocityTargetSpecify=off  VelocityTargetPriority=High  VelocityTargetValue=0  VelocityTargetValueUnits=deg/s
  Revolute Joint D : sm_lib/Joints/Revolute Joint  JointMode=Normal  SenseConstraintForce=off  SenseConstraintForceX=off  SenseConstraintForceY=off  SenseConstraintForceZ=off  SenseConstraintTorque=off  SenseConstraintTorqueX=off  SenseConstraintTorqueY=off  SenseConstraintTorqueZ=off  SenseTotalForce=off  SenseTotalForceX=off  SenseTotalForceY=off  SenseTotalForceZ=off  SenseTotalTorque=off  SenseTotalTorqueX=off  SenseTotalTorqueY=off  SenseTotalTorqueZ=off  CompositeWrenchDir=FollowerOnBase  CompositeWrenchFrame=BaseFrame  EquilibriumPosition=0  EquilibriumPositionUnits=deg  SpringStiffness=0  SpringStiffnessUnits=N*m/deg  DampingCoefficient=0  DampingCoefficientUnits=N*m/(deg/s)  TorqueActuationMode=ComputedTorque  MotionActuationMode=InputMotion  SensePosition=off  SenseVelocity=off  SenseAcceleration=off  SenseTorqueForce=off  SenseLowerLimitTorqueForce=off  SenseUpperLimitTorqueForce=off  LowerLimitSpecify=off  LowerLimitBound=-90  LowerLimitBoundUnits=deg  LowerLimitStiffness=1e4  LowerLimitStiffnessUnits=N*m/deg  LowerLimitDamping=10  LowerLimitDampingUnits=N*m/(deg/s)  LowerLimitTransitionRegionWidth=0.1  LowerLimitTransitionRegionWidthUnits=deg  UpperLimitSpecify=off  UpperLimitBound=90  UpperLimitBoundUnits=deg  UpperLimitStiffness=1e4  UpperLimitStiffnessUnits=N*m/deg  UpperLimitDamping=10  UpperLimitDampingUnits=N*m/(deg/s)  UpperLimitTransitionRegionWidth=0.1  UpperLimitTransitionRegionWidthUnits=deg  PositionTargetSpecify=off  PositionTargetPriority=High  PositionTargetValue=0  PositionTargetValueUnits=deg  VelocityTargetSpecify=off  VelocityTargetPriority=High  VelocityTargetValue=0  VelocityTargetValueUnits=deg/s
  Rigid Transform : sm_lib/Frames and Transforms/Rigid Transform  TranslationMethod=StandardAxis  TranslationStandardOffset=34  TranslationLengthUnit=in  TranslationStandardAxis=-Y  TranslationCartesianOffset=[0 0 0]  TranslationROffset=0  TranslationROffsetUnits=m  TranslationZOffset=0  TranslationZOffsetUnits=m  TranslationThetaOffset=0  TranslationThetaOffsetUnits=deg  RotationMethod=StandardAxis  RotationAngleUnits=deg  RotationStandardAxis=+X  RotationAngle=90  RotationArbitraryAxis=[0 0 1]  FollAlignAxisA=+X  BaseAlignAxisA=+Y  FollAlignAxisB=+Y  BaseAlignAxisB=+Z  RotationSequenceAxes=FollowerAxes  RotationSequence=XYX  RotationSequenceAngles=[0 0 0]  RotationSequenceAnglesUnits=deg  RotationMatrix=[1 0 0; 0 1 0; 0 0 1]
  Simulink-PS Converter : nesl_utility/Simulink-PS Converter  PhysicalDomain=network_engine_domain  SubClassName=ps_input  LeftPortType=input  RightPortType=output  PseudoPeriodic=off  Frequencies=[]  NoiseDistribution=none  NoiseParameters=[]  Unit=in  AffineConversion=off  FilteringAndDerivatives=filter  SimscapeFilterOrder=2  InputFilterTimeConstant=0.1  UdotUserProvided=1
      settings: SourceProductBaseCode=PW,SS
  Simulink-PS Converter1 : nesl_utility/Simulink-PS Converter  PhysicalDomain=network_engine_domain  SubClassName=ps_input  LeftPortType=input  RightPortType=output  PseudoPeriodic=off  Frequencies=[]  NoiseDistribution=none  NoiseParameters=[]  Unit=deg  AffineConversion=off  FilteringAndDerivatives=filter  SimscapeFilterOrder=2  InputFilterTimeConstant=0.01  UdotUserProvided=1
      settings: SourceProductBaseCode=PW,SS
  Sleeve : Subsystem  mask(Sleeve){L=sleeve.length, R=sleeve.radius, t=sleeve.thickness, rgbShaft=sleeve.colorA, rgbBoot=sleeve.colorUJ, rho=sleeve.density}
      mask prompts: L "Shaft Length (in)"; R "Shaft Radius (in)"; t "Shaft Thickness (in)"; rgbShaft "Shaft Color (RGB)"; rgbBoot "Boot Color (RGB)"; rho "Density (kg/m^3)"
      mask help: This block models a sleeve covering the central shaft of the PTO linkage.
      mask init:
      | bootCS = [2.77 0;2.77 0.22;2.66 0.22;2.66 2.33;3.33 2.33;4.55 4.77;4.77 9.5;4.22 4.77;3.11 2.66;2.44 2.66;2.44 0.33;1.44 0.33;1.44 0];
      | shaftCS = [(R-t) -L/2; R -L/2; R L/2; (R-t) L/2];
      mask Display: image(fullfile(matlabroot, 'toolbox', 'physmod', 'sm', 'smdemos', 'pto_shaft', 'images', 'uj_sleeve.png'));
  W : PMIOPort  Side=Left
  tag scope: wu=global
  wires:
  qb/1 -> Simulink-PS Converter/1
  qs/1 -> Simulink-PS Converter1/1
  PS-Simulink Converter/1 -> [wu]
  connections:
  Cylindrical Joint/LConn1 -- Rigid Transform/RConn1 -- Clamp/RConn1
  Rigid Transform/LConn1 -- W/RConn1 -- Base Plate/LConn1
  Cylindrical Joint/RConn1 -- Sleeve/LConn1 -- PTO Linkage/RConn2
  Base Plate/RConn1 -- Revolute Joint A/LConn1
  Simulink-PS Converter1/RConn1 -- Revolute Joint D/LConn2
  Linear Actuator/LConn1 -- Simulink-PS Converter/RConn1
  Base Plate/LConn2 -- Revolute Joint D/LConn1
  Revolute Joint C/RConn1 -- End Plate/LConn1
  Revolute Joint B/RConn1 -- End Plate/RConn1
  PTO Linkage/LConn1 -- Revolute Joint C/LConn1
  Linear Actuator/LConn2 -- Revolute Joint A/RConn1
  PS-Simulink Converter/LConn1 -- Revolute Joint C/RConn2
  Linear Actuator/RConn1 -- Revolute Joint B/LConn1
  Revolute Joint D/RConn1 -- PTO Linkage/RConn1

== system sm_pto_shaft/Bending Motion Input/Nondimensional Actuator Stroke ==
  Demux : Demux  Tag=STV Demux  Outputs=1
      settings: DisplayOption=none
  FromWs : FromWorkspace  Tag=STV FromWs  VariableName=tuvar
      SigBuilderData=|
      | common.afterFinalStr = 'Extrapolate'
      | common.sampleTime = 0
      | dataSet.timeRange = [0 20]
      | dataSet.name = 'Group 1'
      | sbobj.Groups.Name = 'Group 1'
      | sbobj.Groups.Signals.Name = 'Signal 1'
      | sbobj.Groups.Signals.XData = [0 4 4.5 8.5 9 13 13.5 20]
      | sbobj.Groups.Signals.YData = [0 0 -0.5 -0.5 -0.85 -0.85 -1 -1]
      | sbobj.Groups.TimeRange = [0 20]
  Signal 1 : Outport  Tag=STV Outport  VectorParamsAs1DForOutWhenUnconnected=off
  wires:
  Demux/1 -> Signal 1/1
  FromWs/1 -> Demux/1
